simulink model "lab1_2"  (R2022a)
settings: Solver=VariableStepAuto  StartTime=0.0  StopTime=10.0  RelTol=1e-3
settings Model: Creator=Paulo  LastModifiedBy=Paulo

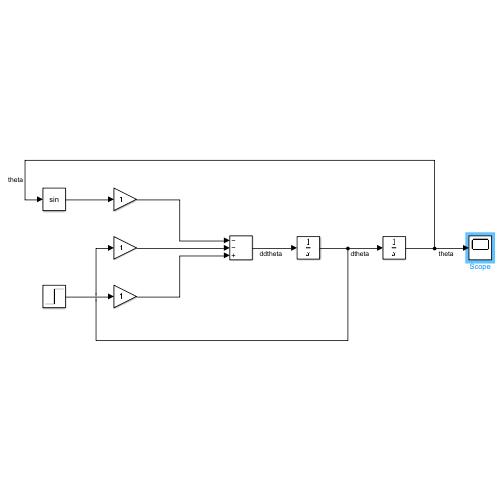
[thumbnail: Simulink's stored preview of the top-level diagram]
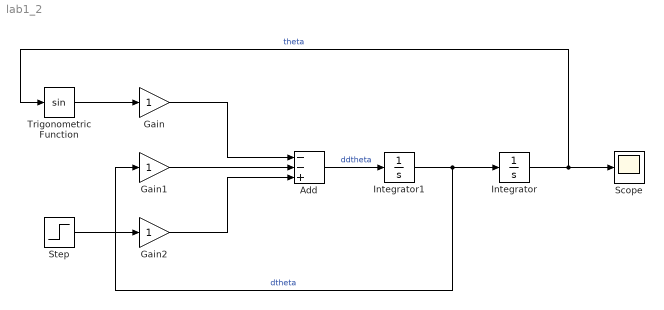
== system lab1_2 ==
  Add : Sum  Inputs=--+
  Gain : Gain
  Gain1 : Gain
  Gain2 : Gain
  Integrator : Integrator
  Integrator1 : Integrator
  Scope : Scope
  Step : Step  SampleTime=0
  Trigonometric Function : Trigonometry
  wires:
  Step/1 -> Gain2/1
  Trigonometric Function/1 -> Gain/1
  Gain/1 -> Add/1
  Gain1/1 -> Add/2
  Gain2/1 -> Add/3
  Add/1 -> Integrator1/1  "ddtheta"
  Integrator1/1 -> Gain1/1, Integrator/1  "dtheta"
  Integrator/1 -> Trigonometric Function/1, Scope/1  "theta"
